simulink model "coupled_tanks_quick_start"  (Simulink 8.3)
settings: Solver=ode1  StartTime=0.0  StopTime=inf  FixedStep=0.1  RelTol=1e-3
PostLoadFcn:
  | qc_set_target_type(getConfigSet(bdroot, 'QUARC Default Target Configuration'));
undefined symbols (not defined in the file): HIL
libraries: quarc_library x3
settings Model: Creator=MLevis  LastModifiedBy=Aluno  SimulationMode=external  ExtModeTrigDuration=30000
settings SolverCC: PositivePriorityOrder=on
settings OptimizationCC: ExpressionDepthLimit=2147483647  InitFltsAndDblsToZero=on
settings DebuggingCC: SaveWithParameterizedLinksMsg=none  MultiTaskDSMMsg=warning  MultiTaskCondExecSysMsg=none  FcnCallInpInsideContextMsg=UseLocalSettings
settings RTWCC: SystemTargetFile=quarc_win64.tlc  TemplateMakefile=quarc_default_tmf  Description=QUARC Win64 Target  ProcessScript=quarc_win64_make_rtw_hook
settings STFCustomTargetCC: TargetPreCompLibLocation=C:\PROGRA~3\QUARC\lib\2014a\win64\release  ConcurrentExecutionCompliant=on  GeneratePreprocessorConditionals=Disable all  CPPClassGenCompliant=on  SystemTargetFile=quarc_win64.tlc
settings GRTTargetCC: TargetPreCompLibLocation=C:\PROGRA~3\QUARC\lib\2014a\win64\release  ParMdlRefBuildCompliant=off  CompOptLevelCompliant=off  MatFileLogging=off  ExtMode=on  ExtModeMexFile=quarc_comm

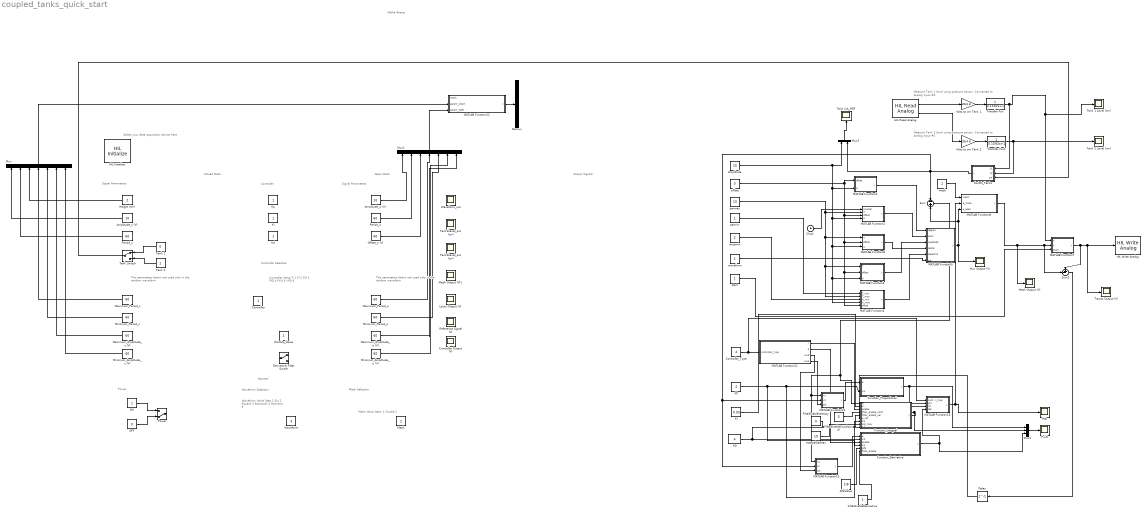
== system coupled_tanks_quick_start ==
  note: Output Signals
  note: Controller
      | Value
      |
      | P
      | 1
      |
      | PI
      | 2
      |
      | PD
      | 3
      |
      | PID
      | 4
      |
      | PI-D
      | 5
      |
      | I-PD
      | 6
  note: Controller Selection
  note: Signal Parameters
  note: Mesh
      | Value
      |
      | Open
      | 1
      |
      | Closed
      | 2
  note: Mesh Selection
  note: Power
  note: Waveform
      | Value
      |
      | Step
      | 1
      |
      | Sin
      | 2
      |
      | Square
      | 3
      |
      | Sawtooth
      | 4
      |
      | Ramdom
      | 5
  note: Waveform Selection
  note: General
  note: Controller
  note: The parameters below are used only in the random waveform
  note: Closed Mesh
  note: Malha Aberta
  note: Measure Tank 2 level using pressure sensor.
      | Connected to Analog Input #1
  note: Measure Tank 1 level using pressure sensor.
      | Connected to Analog Input #0
  note: Select your data acquisition device here
  note: Signal Parameters
  note: The parameters below are used only in the random waveform
  note: Open Mesh
  AlfaValue : Constant  Value=1/8
  "Amplitude " : Constant  Value=15
  Amplitude_c (V) : Constant  Value=10
  Amplitude_o (V) : Constant  Value=10
  Clock : Clock
  Controller : Constant
  Controller Output (V) : Scope
      settings: TimeRange=10  YMin=2.5  YMax=10  SaveName=meshoutput4
  Controller_Type : Constant  Value=4
  Delay : Delay  DelayLength=1  InitialCondition=0
  Demux : Demux  Outputs=7
  Derivative Filter Switch : ManualSwitch
  FilterEnableConditional : Constant  Value=0
  FilterEnableDerivative : Constant
  "FilterEnableVelocity " : Constant  Value=0
  Function_Derivative : MATLAB Function  TreatAsAtomicUnit=on
  Function_Integral : MATLAB Function  TreatAsAtomicUnit=on
  Function_Proportional : MATLAB Function  TreatAsAtomicUnit=on
  HIL Initialize : quarc_library/Data Acquisition/Generic/Configuration/HIL Initialize  object_name=HIL-1  board_type=q2_usb  board_number=0  board_options=d0=digital;d1=digital;led=auto;update_rate=normal;decimation=1  exclusive=off  active=off  hardware_clocks=[0]  clock_modes=[]  initial_clock_frequencies=[]  set_clock_params_at_start=off  set_clock_params_at_switch_in=off  set_clock_frequencies_at_start=off  set_clock_frequencies_at_switch_in=off  analog_input_channels=[0:1]  analog_input_maximums=10  analog_input_minimums=-10  set_analog_input_params_at_start=on  set_analog_input_params_at_switch_in=off  analog_output_channels=[0:1]  analog_output_maximums=10  analog_output_minimums=-10  initial_analog_outputs=[0]  final_analog_outputs=[0]  watchdog_analog_outputs=0  set_analog_output_params_at_start=on  set_analog_output_params_at_switch_in=off  set_analog_outputs_at_start=on  set_analog_outputs_at_switch_in=off  set_analog_outputs_at_terminate=on  set_analog_outputs_at_switch_out=off  set_analog_outputs_on_watchdog=off  digital_input_channels=[]  digital_output_channels=[]  digital_output_configuration=[]  initial_digital_outputs=[1]  final_digital_outputs=[1]  watchdog_digital_outputs=[1]  set_digital_output_params_at_start=off  set_digital_output_params_at_switch_in=off  set_digital_outputs_at_start=on  set_digital_outputs_at_switch_in=off  set_digital_outputs_at_terminate=on  set_digital_outputs_at_switch_out=off  set_digital_outputs_on_watchdog=off  encoder_channels=[0:1]  quadrature=[4]  encoder_filter_frequency=[]  initial_encoder_counts=[0]  set_encoder_params_at_start=on  set_encoder_params_at_switch_in=off  set_encoder_counts_at_start=on  set_encoder_counts_at_switch_in=off  pwm_channels=[]  pwm_modes=[0]  pwm_frequency=1/0.020  pwm_configuration=[]  pwm_alignment=[]  pwm_polarity=[]  pwm_leading_deadband=[]  pwm_trailing_deadband=[]  initial_pwm_outputs=[0]  final_pwm_outputs=[0]  watchdog_pwm_outputs=[0]  set_pwm_params_at_start=on  set_pwm_params_at_switch_in=off  set_pwm_outputs_at_start=on  set_pwm_outputs_at_switch_in=off  set_pwm_outputs_at_terminate=on  set_pwm_outputs_at_switch_out=off  set_pwm_outputs_on_watchdog=off  other_output_channels=[]  initial_other_outputs=[]  final_other_outputs=[]  watchdog_other_outputs=[]  set_other_outputs_at_start=off  set_other_outputs_at_switch_in=off  set_other_outputs_at_terminate=off  set_other_outputs_at_switch_out=off  set_other_outputs_on_watchdog=off
  HIL Read Analog : quarc_library/Data Acquisition/Generic/Immediate I//O/HIL Read Analog  object_name=HIL-1  channels=[0:1]  sample_time=qc_get_step_size  active=on  vector_output=off
  HIL Write Analog : quarc_library/Data Acquisition/Generic/Immediate I//O/HIL Write Analog  object_name=HIL-1  channels=0  sample_time=-1  active=off  vector_input=off
  Height (cm) : Constant  Value=2
  IntegralSatMax : Constant  Value=10
  KD : Constant  Value=4
  KI : Constant  Value=0.05
  KP : Constant  Value=2
  Kd : Constant
  Ki : Constant
  Kp : Constant
  Locks Output (V) : Scope
      settings: TimeRange=10  YMin=2.5  YMax=10  SaveName=meshoutput2
  MATLAB Function1 : MATLAB Function  TreatAsAtomicUnit=on
  MATLAB Function11 : MATLAB Function  TreatAsAtomicUnit=on
  MATLAB Function12 : MATLAB Function  TreatAsAtomicUnit=on
  MATLAB Function13 : MATLAB Function  TreatAsAtomicUnit=on
  MATLAB Function14 : MATLAB Function  TreatAsAtomicUnit=on
  MATLAB Function16 : MATLAB Function  TreatAsAtomicUnit=on
  MATLAB Function2 : MATLAB Function  TreatAsAtomicUnit=on
  MATLAB Function3 : MATLAB Function  TreatAsAtomicUnit=on
  MATLAB Function4 : MATLAB Function  TreatAsAtomicUnit=on
  MATLAB Function5 : MATLAB Function  TreatAsAtomicUnit=on
  MATLAB Function6 : MATLAB Function  TreatAsAtomicUnit=on
  MATLAB Function7 : MATLAB Function  TreatAsAtomicUnit=on
  MATLAB Function8 : MATLAB Function  TreatAsAtomicUnit=on
  Maximum_Amplitude_c (V) : Constant  Value=60
  Maximum_Amplitude_o (V) : Constant  Value=60
  Maximum_Period_c : Constant  Value=60
  Maximum_Period_o : Constant  Value=60
  Mesh : Constant  Value=2
  Mesh Output (V) : Scope
      settings: TimeRange=100  YMin=0  YMax=30  SaveName=meshoutput
  Mesh Output (V)1 : Scope
      settings: TimeRange=10  YMin=2.5  YMax=10  SaveName=meshoutput1
  Minimum_Amplitude_c (V) : Constant  Value=60
  Minimum_Amplitude_o (V) : Constant  Value=60
  Minimum_Period_c : Constant  Value=60
  Minimum_Period_o : Constant  Value=60
  Mux : Mux  Inputs=7
  Mux Output (V) : Scope
      settings: TimeRange=100  SaveName=muxoutput
  Mux1 : Mux  Inputs=7
  Mux2 : Mux  Inputs=3
  Mux3 : Mux  Inputs=2
  OFF : Constant  Value=0
  ON : Constant
  Offset_o (V) : Constant  Value=60
  P-I-D : Scope
      settings: ShowLegends=on  TimeRange=100  YMin=-100  YMax=100  SaveName=PID
  PID : Scope
      settings: TimeRange=100  YMin=0  YMax=100
  Period_c : Constant  Value=60
  Period_o : Constant  Value=60
  Power : ManualSwitch  CurrentSetting=0
  Reference Signal (V) : Scope
      settings: TimeRange=10  YMin=2.5  YMax=10  SaveName=meshoutput3
  Sum : Sum  Inputs=-+
  Sum1 : Sum  Inputs=+-|
  Switch_Tanks : MATLAB Function  TreatAsAtomicUnit=on
  Tank 1 : Constant  Value=0
  Tank 1 Level (cm) : Scope
      settings: TimeRange=100  YMin=0  YMax=30  SaveName=tank1level
  Tank 2 : Constant
  Tank 2 Level (cm) : Scope
      settings: TimeRange=300  YMin=-1  YMax=30  SaveName=tank2level
  Tank LVL_REF : Scope
      settings: ShowLegends=on  TimeRange=300  YMin=0  YMax=30  SaveName=tank1level1
  Tank Switch : ManualSwitch
  Tank1Level_out (cm) : Scope
      settings: TimeRange=10  YMin=4.125  YMax=4.5  SaveName=muxoutput2
  Tank2Level_out (cm) : Scope
      settings: TimeRange=10  YMin=4.125  YMax=4.5  SaveName=muxoutput3
  Transfer Fcn : TransferFcn  Denominator=[0.1592 1]
  Transfer Fcn1 : TransferFcn  Denominator=[0.1592 1]
  Travas Output (V) : Scope
      settings: TimeRange=100  SaveName=travaoutput
  "Volts to cm Tank 1 " : Gain  Gain=30/4.8
  Volts to cm Tank 2 : Gain  Gain=30/4.8
  Waveform : Constant  Value=3
  Waveform_out : Scope
      settings: TimeRange=10  YMin=4.125  YMax=4.5  SaveName=muxoutput1
  WindUp_Value : Constant
  ampmin : Constant  Value=2
  mesh : Constant  Value=2
  offset : Constant  Value=0
  permax : Constant  Value=10
  permin : Constant
  start : Constant
  waveform : Constant
  wires:
  MATLAB Function2/1(y) -> MATLAB Function5/1(degrau)
  MATLAB Function1/1(y) -> MATLAB Function5/2(seno)
  MATLAB Function6/1(y) -> MATLAB Function5/4(dente)
  MATLAB Function3/1(y) -> MATLAB Function5/3(quadrada)
  MATLAB Function4/1(y) -> MATLAB Function5/5(aleatoria)
  offset/1 -> MATLAB Function2/1(offset), MATLAB Function1/3(offset), MATLAB Function4/5(offset), MATLAB Function3/2(offset), MATLAB Function6/2(offset)
  permax/1 -> MATLAB Function4/2(T_max), MATLAB Function3/1(T), MATLAB Function6/1(T), MATLAB Function1/2(T)
  Transfer Fcn/1 -> Switch_Tanks/1(x1), MATLAB Function7/1(h), Tank 1 Level (cm)/1
  waveform/1 -> MATLAB Function5/6(sel)
  permin/1 -> MATLAB Function4/1(T_min)
  ampmin/1 -> MATLAB Function4/3(A_min)
  start/1 -> MATLAB Function7/3(start)
  Clock/1 -> MATLAB Function1/1(counter)
  HIL Read Analog/1 -> "Volts to cm Tank 1 "/1
  "Volts to cm Tank 1 "/1 -> Transfer Fcn/1
  Transfer Fcn1/1 -> Switch_Tanks/2(x2), Tank 2 Level (cm)/1
  Volts to cm Tank 2/1 -> Transfer Fcn1/1
  HIL Read Analog/2 -> Volts to cm Tank 2/1
  "Amplitude "/1 -> Mux3/1, MATLAB Function1/4(A), MATLAB Function6/3(A), MATLAB Function3/3(A), MATLAB Function4/4(A_max), MATLAB Function2/2(A)
  MATLAB Function7/1(y) -> Sum1/1, HIL Write Analog/1, Travas Output (V)/1
  mesh/1 -> MATLAB Function8/1(mesh)
  MATLAB Function5/1(y) -> Mux Output (V)/1, Sum/2, MATLAB Function8/3(a_open)
  MATLAB Function8/1(y) -> Mesh Output (V)/1, Sum1/2, MATLAB Function7/2(u)
  ON/1 -> Power/1
  OFF/1 -> Power/2
  Tank 1/1 -> Tank Switch/1
  Tank 2/1 -> Tank Switch/2
  Function_Proportional/1(y) -> MATLAB Function16/2(pro), Mux2/1
  Function_Integral/1(y) -> MATLAB Function16/3(int), Mux2/2
  Sum/1 -> MATLAB Function14/1(x1), MATLAB Function13/1(x1), Function_Integral/1(e)
  MATLAB Function11/1(i) -> Function_Integral/3(enable)
  KP/1 -> Function_Derivative/4(Kp), Function_Integral/7(Kp), Function_Proportional/2(Kp)
  MATLAB Function11/2(d) -> Function_Derivative/3(enable)
  Controller_Type/1 -> MATLAB Function16/1(control_type), MATLAB Function11/1(controller_type)
  MATLAB Function16/1(y) -> MATLAB Function8/2(a_close), PID/1
  Amplitude_o (V)/1 -> Mux1/1
  Period_o/1 -> Mux1/2
  Offset_o (V)/1 -> Mux1/3
  Maximum_Period_o/1 -> Mux1/4
  Mux2/1 -> P-I-D/1
  Minimum_Period_o/1 -> Mux1/5
  Maximum_Amplitude_o (V)/1 -> Mux1/6
  Minimum_Amplitude_o (V)/1 -> Mux1/7
  Mux1/1 -> MATLAB Function12/3(param_open)
  Mux/1 -> MATLAB Function12/2(param_close)
  MATLAB Function12/1(y) -> Demux/1
  Height (cm)/1 -> Mux/3
  Amplitude_c (V)/1 -> Mux/1
  Period_c/1 -> Mux/2
  Maximum_Period_c/1 -> Mux/4
  Minimum_Period_c/1 -> Mux/5
  Maximum_Amplitude_c (V)/1 -> Mux/6
  Minimum_Amplitude_c (V)/1 -> Mux/7
  MATLAB Function13/1(y) -> Function_Derivative/1(e)
  MATLAB Function11/3(swd) -> MATLAB Function13/3(sel)
  Switch_Tanks/1(y) -> Mux3/2, Sum/1, MATLAB Function14/2(x2), MATLAB Function13/2(x2)
  MATLAB Function14/1(y) -> Function_Proportional/1(e)
  MATLAB Function11/4(swp) -> MATLAB Function14/3(sel)
  Tank Switch/1 -> Switch_Tanks/3(sel)
  Mux3/1 -> Tank LVL_REF/1
  FilterEnableConditional/1 -> Function_Integral/4(filter_enable_cond)
  KD/1 -> Function_Integral/9(Kd), Function_Derivative/2(Kd)
  Function_Derivative/1(y) -> MATLAB Function16/4(der), Mux2/3
  AlfaValue/1 -> Function_Derivative/5(alfa)
  FilterEnableDerivative/1 -> Function_Derivative/6(filter_enable)
  "FilterEnableVelocity "/1 -> Function_Integral/5(filter_enable_vel)
  KI/1 -> Function_Integral/2(Ki)
  Delay/1 -> Function_Integral/6(e_sat)
  Sum1/1 -> Delay/1
  IntegralSatMax/1 -> Function_Integral/8(sat_max)

== matlab function MATLAB Function1 ==
  data: counter input double; y output double; T input double; offset input double; A input double
function y = seno(counter, T, offset, A)

%counter = cast(counter, 'double');

y = A*sin(counter*2*pi/T) + offset;

== matlab function MATLAB Function2 ==
  data: offset input double; y output double; A input double
function y = degrau(offset, A)



y = A + offset;

== matlab function MATLAB Function6 ==
  data: y output double; T input double; offset input double; A input double
function y = dente(T, offset, A)

persistent counter_d;

if isempty(counter_d)
   counter_d = 0; 
end


y = counter_d*A*2/(10*T) + offset - A;

counter_d = counter_d + 1;

if (counter_d > T*10)
   counter_d = 0;
end

== matlab function MATLAB Function3 ==
  data: y output double; T input double; offset input double; A input double
function y = quadrada(T, offset, A)

persistent counter_q;

if isempty(counter_q)
   counter_q = 0; 
end

counter_q = counter_q + 1;

if (counter_q <= 5*T)
    y = -A + offset;
elseif (counter_q > 5*T)
    y = A + offset;
else
    y = 0;
end

if (counter_q >= 10*T)
   counter_q = 0; 
end

== matlab function MATLAB Function4 ==
  data: T_min input double; y output double; T_max input double; A_min input double; A_max input double; offset input double
function y = aleatoria(T_min, T_max, A_min, A_max, offset)

persistent T_now;
persistent A_now;
persistent counter_a;

if isempty(counter_a)
    T_now = T_min + (T_max - T_min)*rand;
    A_now = A_min + (A_max - A_min)*rand + offset;
    counter_a = 0;
end

counter_a = counter_a + 1;

y = A_now;

if (counter_a >= T_now*10)
    T_now = T_min + (T_max - T_min)*rand;
    A_now = A_min + (A_max - A_min)*rand + offset;
    counter_a = 0;
end

== matlab function MATLAB Function5 ==
  data: degrau input double; y output double; seno input double; quadrada input double; dente input double; aleatoria input double; sel input double
function y = mux(degrau, seno, quadrada, dente, aleatoria, sel)

switch sel
    case 1
        y = degrau;
    case 2
        y = seno;
    case 3
        y = quadrada;
    case 4
        y = dente;
    case 5
        y = aleatoria;
    otherwise
        y = 0;
end

== matlab function MATLAB Function7 ==
  data: h input double; u input double; y output double; start input double
    function y = travas(h, u, start)
%#codegen
h_max = 30;

%Trava de tensão
if(u < -4)
    u = -4;
end
if(u > 4)
    u = 4;
end

%Trava pra não sugar ar
if(u < 0 & h < 2)
    u = 0;
end

%Trava de transbordamento
% if(h >= h_max - 1.0 & h < h_max - 0.75)
%    u = 0.95*u;
% elseif(h >= h_max - 0.75 & h < h_max - 0.5)
%     u = 0.93*u;
% elseif(h >= h_max - 0.5 & h < h_max - 0.25)
%     u = 0.91*u;
% elseif(h >= h_max - 0.25 & h < h_max)
%     u = 0.88*u;
% elseif(h >= h_max)
%     u = 0;
% end

%
if h >= (h_max-1)
    u = (h_max - h)*u;
end

%
% persistent goingup
% 
% if isempty(goingup)
%    goingup = 1; 
% end
% 
% if goingup == 1
%    if h >= 29
%       u = 0;
%       goingup = 0;
%    end
% else
%     if h <= 25
%        goingup = 1; 
%     else
%        u = 0; 
%     end
% end
    
y = start*u;

== matlab function Function_Proportional ==
  data: e input double; y output double; Kp input double
function y = proportional(e, Kp)

y = Kp*e;

== matlab function MATLAB Function8 ==
  data: mesh input double; a_close input double; y output double; a_open input double
function y = sel_mesh(mesh, a_close, a_open)
%#codegen

if(mesh == 1)
    y = a_open;
else
    y = a_close;
end

== matlab function Function_Integral ==
  data: e input double; y output double; Ki input double; enable input double; filter_enable_cond input double; filter_enable_vel input double; e_sat input double; Kp input double; sat_max input double; Kd input double
function y = integral(e, Ki, enable, filter_enable_cond, filter_enable_vel, e_sat, Kp, sat_max, Kd)

persistent sum;

if isempty(sum)
   sum = 0; 
end

Ti = Kp/Ki;
Td = Kd/Kp;

Tt = sqrt(Ti * Td);

Tt_value = (1/Tt) * e_sat;

if(filter_enable_cond == 1 && sum > sat_max) 
    sum = 0;
elseif(filter_enable_vel == 1)
    sum =  ((Ki*e) + Tt_value)*0.1 + sum;
else
    sum = sum + Ki*e*0.1;
end
y = sum*enable;

== matlab function Function_Derivative ==
  data: e input double; y output double; Kd input double; enable input double; Kp input double; alfa input double; filter_enable input double
function y = derivative(e, Kd, enable, Kp, alfa, filter_enable)

persistent prev_error;
persistent y_error;
persistent aux;

if isempty(prev_error)
   prev_error = 0; 
end

if isempty(y_error)
   y_error = 0; 
end

if isempty(aux)
   aux = 0; 
end


%1/0.1 == 10
Td = Kd/Kp;


if(filter_enable == 1)
    y = ((e - prev_error + alfa*y_error) * Kd)/(1+(Td*alfa));
else
    y = Kd*(e - prev_error)*enable/0.1;
end


prev_error = e;
y_error = y;

end

== matlab function MATLAB Function11 ==
  data: controller_type input double; i output double; d output double; swd output double; swp output double
function [i,d,swd,swp]= fcn(controller_type)

if(controller_type == 1)
    i = 0;
    d = 0;
    swd = 0;
    swp = 0;
elseif(controller_type == 2)
    i = 1;
    d = 0;
    swd = 0;
    swp = 0;
elseif(controller_type == 3)
    i = 0;
    d = 1;
    swd = 0;
    swp = 0;
elseif(controller_type == 4)
    i = 1;
    d = 1;
    swd = 0;
    swp = 0;
elseif(controller_type == 5)
    i = 1;
    d = 1;
    swd = 1;
    swp = 0;
elseif(controller_type == 6)
    i = 1;
    d = 1;
    swd = 1;
    swp = 1;
else
    i = 0;
    d = 0;
    swd = 0;
    swp = 0;
end

== matlab function MATLAB Function12 ==
  data: mesh input double; param_close input double; y output double; param_open input double
function y = param_sw(mesh, param_close, param_open)

if(mesh == 1)
    y = param_open;
else
    y = param_close;
end

== matlab function MATLAB Function13 ==
  data: x1 input double; x2 input double; y output double; sel input double
function y = switch_deriv(x1, x2, sel)

if sel == 0
    y = x1; 
else
    y = x2;
end
    
end

== matlab function MATLAB Function14 ==
  data: x1 input double; x2 input double; y output double; sel input double
function y = switch_prop(x1, x2, sel)

if sel == 0
    y = x1; 
else
    y = x2;
end
    
end

== matlab function Switch_Tanks ==
  data: x1 input double; x2 input double; y output double; sel input double
function y = switch2(x1, x2, sel)

if sel == 0
    y = x1; 
else
    y = x2;
end
    
end

== matlab function MATLAB Function16 ==
  data: control_type input double; y output double; pro input double; int input double; der input double
function y = adding(control_type, pro, int, der)
%#codegen

if(control_type >= 1 && control_type <= 4)
   y = pro + int + der;
elseif(control_type == 5)
    y = pro + int - der;
else
    y = int - pro - der;
end
